simulink model "sf_temporal_logic_scheduler_with_sl_fcns"  (R2017b)
settings: Solver=FixedStepDiscrete  StartTime=0.0  StopTime=5  RelTol=1e-3  EnableMultiTasking=on
model workspace (MAT data in the model file):
  deltat = 0.001
settings Model: Creator=The MathWorks, Inc.  LastModifiedBy=The MathWorks, Inc.
settings SolverCC: InsertRTBMode=Auto
settings DataIOCC: LimitDataPoints=on  SaveFormat=Array
settings OptimizationCC: ExpressionDepthLimit=2147483647  InitFltsAndDblsToZero=on  EfficientMapNaN2IntZero=off  LifeSpan=inf
settings DebuggingCC: SaveWithParameterizedLinksMsg=none  UnderspecifiedInitializationDetection=Classic  MergeDetectMultiDrivingBlocksExec=none  SignalResolutionControl=TryResolveAllWithWarning  SolverPrmCheckMsg=warning  InheritedTsInSrcMsg=none  MultiTaskDSMMsg=warning  MultiTaskCondExecSysMsg=none  FcnCallInpInsideContextMsg=warning  StateNameClashWarn=warning  StrictBusMsg=None  SFUnexpectedBacktrackingDiag=warning  SFNoUnconditionalDefaultTransitionDiag=warning  SFExecutionAtInitializationDiag=none
settings HardwareCC: ProdBitPerPointer=32  ProdBitPerSizeT=32  ProdBitPerPtrDiffT=32  ProdLargestAtomicFloat=None  ProdIntDivRoundTo=Undefined  ProdEndianess=Unspecified  ProdWordSize=32  ProdHWDeviceType=32-bit Generic
settings ModelReferenceCC: PropagateSignalLabelsOutOfModel=off
settings SFSimCC: SFSimEcho=off  SimParseCustomCode=off
settings CodeAppCC: StateflowObjectComments=on
settings GRTTargetCC: TargetFcnLib=ansi_tfl_tmw.mat  TargetLangStandard=C89/C90 (ANSI)  GeneratePreprocessorConditionals=Disable all  CombineOutputUpdateFcns=off  GRTInterface=on
settings ConfigComp: CovMetricSettings=dw  CovHtmlReporting=on  CovSaveCumulativeToWorkspaceVar=on  CovSaveSingleToWorkspaceVar=on  CovExternalEMLEnable=off  CovSFcnEnable=off

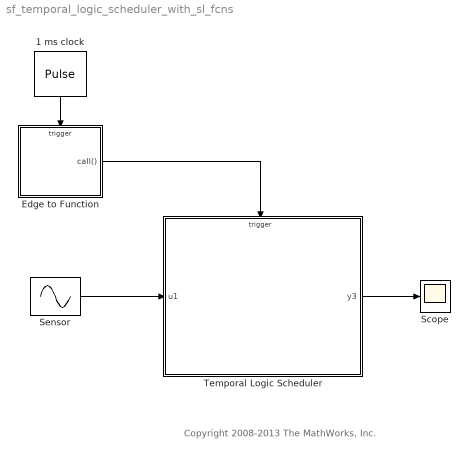
== system sf_temporal_logic_scheduler_with_sl_fcns ==
  note: Copyright 2008-2013 The MathWorks, Inc.
  1 ms clock : DiscretePulseGenerator  PulseType=Time based  Period=0.001  PulseWidth=10
  "Edge to Function " : Stateflow chart  TreatAsAtomicUnit=on
  Scope : Scope
  Sensor : Sin  Frequency=40  Phase=-pi/8
  Temporal Logic Scheduler : Stateflow chart  TreatAsAtomicUnit=on
  wires:
  Sensor/1 -> Temporal Logic Scheduler/1(u1)
  1 ms clock/1 -> "Edge to Function "/Trigger
  "Edge to Function "/1(call()) -> Temporal Logic Scheduler/Trigger
  Temporal Logic Scheduler/1(y3) -> Scope/1

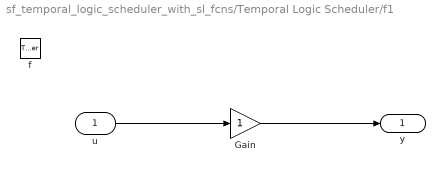
== system sf_temporal_logic_scheduler_with_sl_fcns/Temporal Logic Scheduler/f1 ==
  u : Inport
  f : TriggerPort  TriggerType=function-call  VariantControl=(inherit)
      settings: CopyFcn=Stateflow.SLINSF.SimulinkMan.removeBlockPreDeleteFcn  PreDeleteFcn=Stateflow.SLINSF.SimulinkMan.unsafePredeleteFcn
  Gain : Gain
  y : Outport
  wires:
  u/1 -> Gain/1
  Gain/1 -> y/1

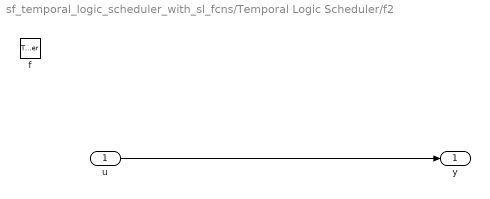
== system sf_temporal_logic_scheduler_with_sl_fcns/Temporal Logic Scheduler/f2 ==
  u : Inport
  f : TriggerPort  TriggerType=function-call  VariantControl=(inherit)
      settings: CopyFcn=Stateflow.SLINSF.SimulinkMan.removeBlockPreDeleteFcn  PreDeleteFcn=Stateflow.SLINSF.SimulinkMan.unsafePredeleteFcn
  y : Outport  InitialOutput=0
  wires:
  u/1 -> y/1

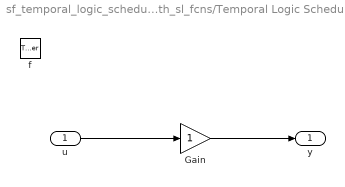
== system sf_temporal_logic_scheduler_with_sl_fcns/Temporal Logic Scheduler/f3 ==
  u : Inport
  f : TriggerPort  TriggerType=function-call  VariantControl=(inherit)
      settings: CopyFcn=Stateflow.SLINSF.SimulinkMan.removeBlockPreDeleteFcn  PreDeleteFcn=Stateflow.SLINSF.SimulinkMan.unsafePredeleteFcn
  Gain : Gain
  y : Outport
  wires:
  u/1 -> Gain/1
  Gain/1 -> y/1

== stateflow chart sf_temporal_logic_scheduler_with_sl_fcns/Temporal Logic Scheduler ==
  state y = f1(u) [function]
  state FastScheduler
    du: y = u1-y2;
    on every(1,call): y1 = f1(y) ;
    on every(2,call): y2 = f2(y1);
    on every(4,call): y3 = f3(y2);
  state y = f2(u) [function]
  state SlowScheduler
    du: y = u1-y2;
    on every(8,call): y1 = f1(y);
    on every(16,call): y2 = f2(y1);
    on every(32,call): y3 = f3(y2);
  state y = f3(u) [function]
  (default) -> FastScheduler
  SlowScheduler -> FastScheduler : after(100,call)
  FastScheduler -> SlowScheduler : after(100,call)
  data: u function_input; y function_output; u function_input; y function_output; u function_input; y function_output; y local double; u1 input; y1 local double; y2 local double; y3 output double
  events: call input FUNCTION_CALL_EVENT

== stateflow chart sf_temporal_logic_scheduler_with_sl_fcns/Edge to Function  ==
  (default) -> (junction 2) : {call;}
  events: edge input RISING_EDGE_EVENT; call output FUNCTION_CALL_EVENT
